simulink model "quadrotor_adaptive_control"  (R2025b)
settings: Solver=ode4  StartTime=0.0  StopTime=150  FixedStep=0.001  MaxStep=1e-3  RelTol=1e-6
values from neighbouring files (symbols this model uses):
  pi_hat0 = [0.899; 0.009; 0.009; 0.015]    [pi_hat_init.m]
undefined symbols (not defined in the file or in its folder): F, Light, MIL
libraries: simulink x5, aerolibwind2 x3
(part 1 of 2)
settings Model: Creator=Marcus  LastModifiedBy=Marcus
settings SolverCC: ZeroCrossAlgorithm=Adaptive
settings DataIOCC: Refine=5
settings DebuggingCC: MaskedZcDiagnostic=none  IgnoredZcDiagnostic=none

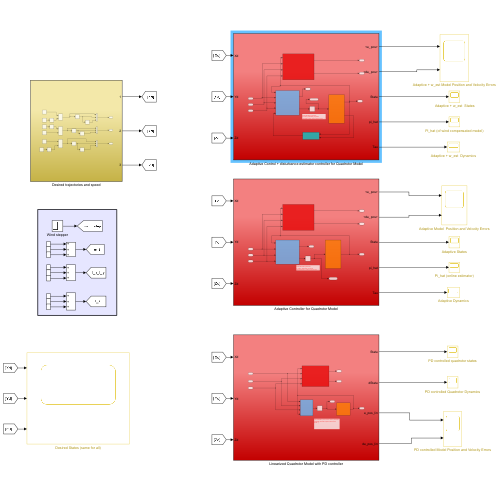
[thumbnail: Simulink's stored preview of the top-level diagram]
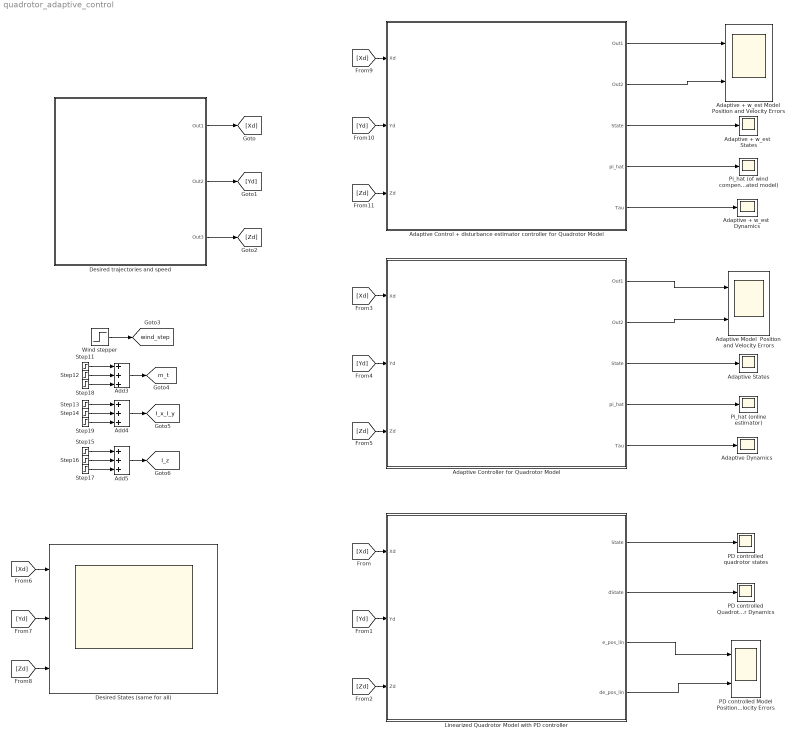
== system quadrotor_adaptive_control ==
  " Adaptive + w_est  States" : Scope
      settings: ActiveDisplayYMinimum=-16.300355765094039  ActiveDisplayYMaximum=35.268121644777928  DataLoggingVariableName=ScopeData9
  Adaptive + w_est  Dynamics : Scope
      settings: ActiveDisplayYMinimum=-3.5572864670508944  ActiveDisplayYMaximum=4.821971659312168  DataLoggingVariableName=ScopeData6
  Adaptive + w_est Model Position and Velocity Errors : Scope  NumInputPorts=2
      settings: ActiveDisplayYMinimum=-0.49516573839944322  ActiveDisplayYMaximum=0.3279252812181247  DataLoggingVariableName=ScopeData7
  Adaptive Control + disturbance estimator controller for Quadrotor Model : Subsystem
  Adaptive Controller for Quadrotor Model : Subsystem
  Adaptive Dynamics : Scope
      settings: ActiveDisplayYMinimum=-0.23880128032010212  ActiveDisplayYMaximum=0.18338732165681021  DataLoggingVariableName=ScopeData2
  Adaptive Model  Position and Velocity Errors : Scope  NumInputPorts=2
      settings: ActiveDisplayYMinimum=-0.24580483450326776  ActiveDisplayYMaximum=0.48785875848156551  DataLoggingVariableName=ScopeData3
  Adaptive States : Scope
      settings: ActiveDisplayYMinimum=-130.48583470390469  ActiveDisplayYMaximum=721.89809496547809
  Add3 : Sum  Inputs=+++
  Add4 : Sum  Inputs=+++
  Add5 : Sum  Inputs=+++
  Desired States (same for all) : Scope  NumInputPorts=3
      settings: ActiveDisplayYMinimum=-80.393154494146742  ActiveDisplayYMaximum=268.39207033687438
  Desired trajectories and speed : Subsystem
  Linearized Quadrotor Model with PD controller : Subsystem
  PD controlled Model Position and Velocity Errors : Scope  NumInputPorts=2
      settings: ActiveDisplayYMinimum=-1.1379166870147581  ActiveDisplayYMaximum=1.3439227788194077  DataLoggingVariableName=ScopeData8
  PD controlled Quadrotor Dynamics : Scope
      settings: ActiveDisplayYMinimum=-12.548402884641092  ActiveDisplayYMaximum=10.307273643056192  DataLoggingVariableName=ScopeData4
  PD controlled quadrotor states : Scope
      settings: ActiveDisplayYMinimum=-85.7969690316985  ActiveDisplayYMaximum=661.47891308235489  DataLoggingVariableName=ScopeData5
  Pi_hat (of wind compensated model) : Scope
      settings: ActiveDisplayYMinimum=1.5892477620700283  ActiveDisplayYMaximum=2.69868157713973  DataLoggingVariableName=pi_hat1  DataLoggingSaveFormat=Array
  Pi_hat (online estimator) : Scope
      settings: ActiveDisplayYMinimum=0.15390009207158523  ActiveDisplayYMaximum=0.19714737045984923  DataLoggingVariableName=pi_hat  DataLoggingSaveFormat=Array
  Step11 : Step  Time=50  Before=0.899  After=0.899+0.8  SampleTime=0
  Step12 : Step  Time=100  After=0.3  SampleTime=0
  Step13 : Step  Time=50  Before=0.009  After=0.009+0.002  SampleTime=0
  Step14 : Step  Time=100  After=0.28e-4  SampleTime=0
  Step15 : Step  Time=50  Before=0.015  After=0.015+0.15e-3*rand  SampleTime=0
  Step16 : Step  Time=100  After=0.2e-3  SampleTime=0
  Step17 : Step  Time=250  After=-0.12e-3  SampleTime=0
  Step18 : Step  Time=300  After=-0.2  SampleTime=0
  Step19 : Step  Time=240  After=-0.08e-4  SampleTime=0
  Wind stepper : Step  Time=85  SampleTime=0
  tag scope: I_x_I_y=global, I_z=global, m_t=global, wind_step=global
  wires:
  Linearized Quadrotor Model with PD controller/1(State) -> PD controlled quadrotor states/1
  Linearized Quadrotor Model with PD controller/2(dState) -> PD controlled Quadrotor Dynamics/1
  [Xd] -> Linearized Quadrotor Model with PD controller/1(Xd)
  [Yd] -> Linearized Quadrotor Model with PD controller/2(Yd)
  [Zd] -> Linearized Quadrotor Model with PD controller/3(Zd)
  [Xd] -> Adaptive Controller for Quadrotor Model/1(Xd)
  [Yd] -> Adaptive Controller for Quadrotor Model/2(Yd)
  [Zd] -> Adaptive Controller for Quadrotor Model/3(Zd)
  Adaptive Controller for Quadrotor Model/4(pi_hat) -> Pi_hat (online estimator)/1
  Adaptive Controller for Quadrotor Model/3(State) -> Adaptive States/1
  Adaptive Controller for Quadrotor Model/5(Tau) -> Adaptive Dynamics/1
  Adaptive Controller for Quadrotor Model/1(Out1) -> Adaptive Model  Position and Velocity Errors/1
  Adaptive Controller for Quadrotor Model/2(Out2) -> Adaptive Model  Position and Velocity Errors/2
  [Xd] -> Desired States (same for all)/1
  [Yd] -> Desired States (same for all)/2
  [Zd] -> Desired States (same for all)/3
  Linearized Quadrotor Model with PD controller/3(e_pos_lin) -> PD controlled Model Position and Velocity Errors/1
  Linearized Quadrotor Model with PD controller/4(de_pos_lin) -> PD controlled Model Position and Velocity Errors/2
  Adaptive Control + disturbance estimator controller for Quadrotor Model/5(Tau) -> Adaptive + w_est  Dynamics/1
  Adaptive Control + disturbance estimator controller for Quadrotor Model/4(pi_hat) -> Pi_hat (of wind compensated model)/1
  Adaptive Control + disturbance estimator controller for Quadrotor Model/2(Out2) -> Adaptive + w_est Model Position and Velocity Errors/2
  Adaptive Control + disturbance estimator controller for Quadrotor Model/1(Out1) -> Adaptive + w_est Model Position and Velocity Errors/1
  [Yd] -> Adaptive Control + disturbance estimator controller for Quadrotor Model/2(Yd)
  [Xd] -> Adaptive Control + disturbance estimator controller for Quadrotor Model/1(Xd)
  Adaptive Control + disturbance estimator controller for Quadrotor Model/3(State) -> " Adaptive + w_est  States"/1
  [Zd] -> Adaptive Control + disturbance estimator controller for Quadrotor Model/3(Zd)
  Wind stepper/1 -> [wind_step]
  Step16/1 -> Add5/2
  Step14/1 -> Add4/2
  Step11/1 -> Add3/1
  Step19/1 -> Add4/3
  Add4/1 -> [I_x_I_y]
  Step13/1 -> Add4/1
  Step18/1 -> Add3/3
  Add3/1 -> [m_t]
  Add5/1 -> [I_z]
  Step12/1 -> Add3/2
  Step15/1 -> Add5/1
  Step17/1 -> Add5/3
  Desired trajectories and speed/1(Out1) -> [Xd]
  Desired trajectories and speed/2(Out2) -> [Yd]
  Desired trajectories and speed/3(Out3) -> [Zd]

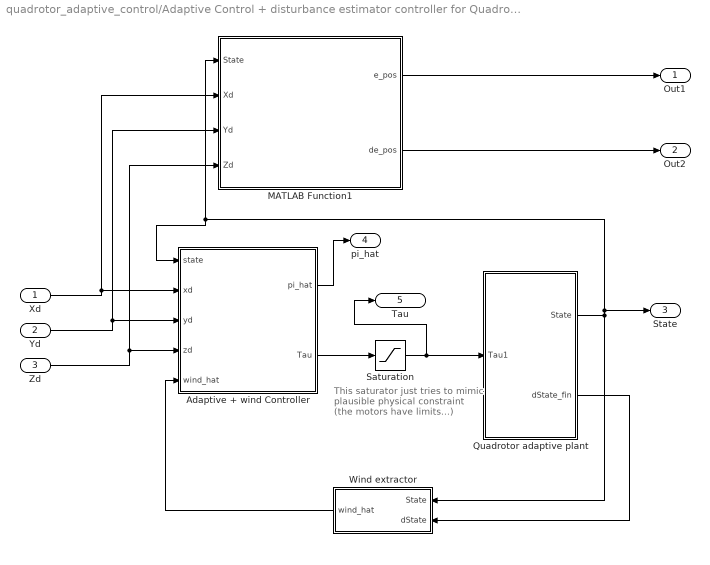
== system quadrotor_adaptive_control/Adaptive Control + disturbance estimator controller for Quadrotor Model ==
  note: This saturator just tries
      | to mimic plausible physical
      | constraint (the motors have limits...)
  Xd : Inport
  Yd : Inport  Port=2
  Zd : Inport  Port=3
  Adaptive + wind Controller : Subsystem
  MATLAB Function1 : MATLAB Function  TreatAsAtomicUnit=on
  Quadrotor adaptive plant : Subsystem
  Saturation : Saturate  UpperLimit=[25;0.8;0.8;0.10]  LowerLimit=[0;-0.8;-0.8;-0.10]
  Wind extractor : Subsystem
  Out1 : Outport
  Out2 : Outport  Port=2
  State : Outport  Port=3
  pi_hat : Outport  Port=4
  Tau : Outport  Port=5
  wires:
  Zd/1 -> MATLAB Function1/4(Zd), Adaptive + wind Controller/4(zd)
  Xd/1 -> MATLAB Function1/2(Xd), Adaptive + wind Controller/2(xd)
  Adaptive + wind Controller/1(pi_hat) -> pi_hat/1
  Yd/1 -> MATLAB Function1/3(Yd), Adaptive + wind Controller/3(yd)
  MATLAB Function1/2(de_pos) -> Out2/1
  MATLAB Function1/1(e_pos) -> Out1/1
  Quadrotor adaptive plant/1(State) -> State/1, MATLAB Function1/1(State), Adaptive + wind Controller/1(state), Wind extractor/1(State)
  Adaptive + wind Controller/2(Tau) -> Saturation/1
  Quadrotor adaptive plant/2(dState_fin) -> Wind extractor/2(dState)
  Wind extractor/1(wind_hat) -> Adaptive + wind Controller/5(wind_hat)
  Saturation/1 -> Tau/1, Quadrotor adaptive plant/1(Tau1)

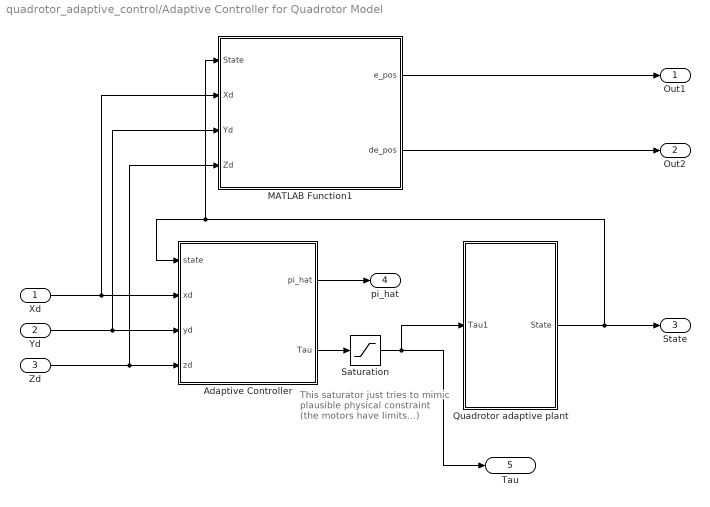
== system quadrotor_adaptive_control/Adaptive Controller for Quadrotor Model ==
  note: This saturator just tries
      | to mimic plausible physical
      | constraint (the motors have limits...)
  Xd : Inport
  Yd : Inport  Port=2
  Zd : Inport  Port=3
  Adaptive Controller : Subsystem
  MATLAB Function1 : MATLAB Function  TreatAsAtomicUnit=on
  Quadrotor adaptive plant : Subsystem
  Saturation : Saturate  UpperLimit=[25;0.8;0.8;0.10]  LowerLimit=[0;-0.8;-0.8;-0.10]
  Out1 : Outport
  Out2 : Outport  Port=2
  State : Outport  Port=3
  pi_hat : Outport  Port=4
  Tau : Outport  Port=5
  wires:
  Zd/1 -> MATLAB Function1/4(Zd), Adaptive Controller/4(zd)
  Adaptive Controller/2(Tau) -> Saturation/1
  Xd/1 -> MATLAB Function1/2(Xd), Adaptive Controller/2(xd)
  Adaptive Controller/1(pi_hat) -> pi_hat/1
  Yd/1 -> Adaptive Controller/3(yd), MATLAB Function1/3(Yd)
  MATLAB Function1/2(de_pos) -> Out2/1
  MATLAB Function1/1(e_pos) -> Out1/1
  Quadrotor adaptive plant/1(State) -> State/1, MATLAB Function1/1(State), Adaptive Controller/1(state)
  Saturation/1 -> Quadrotor adaptive plant/1(Tau1), Tau/1

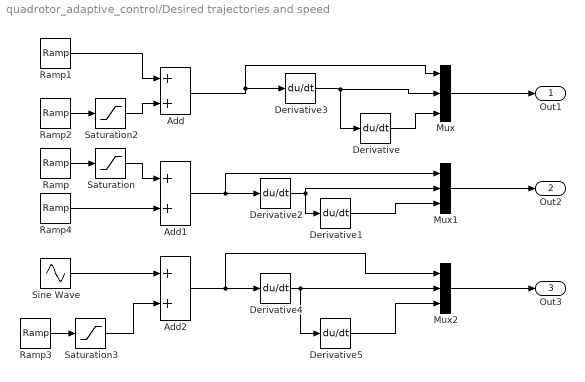
== system quadrotor_adaptive_control/Desired trajectories and speed ==
  Add : Sum
  Add1 : Sum
  Add2 : Sum
  Derivative{,1..5} (6 alike) : Derivative  CoefficientInTFapproximation=1e6
  Mux : Mux  Inputs=3
  Mux1 : Mux  Inputs=3
  Mux2 : Mux  Inputs=3
  Ramp : simulink/Sources/Ramp  slope=1.2  start=0  InitialOutput=0
  Ramp1 : simulink/Sources/Ramp  slope=0.3  start=0  InitialOutput=0
  Ramp2 : simulink/Sources/Ramp  slope=-1.2  start=65  InitialOutput=0
  Ramp3 : simulink/Sources/Ramp  slope=.4  start=70  InitialOutput=0
  Ramp4 : simulink/Sources/Ramp  slope=.2  start=20  InitialOutput=0
  Saturation : Saturate  UpperLimit=15  LowerLimit=0
  Saturation2 : Saturate  UpperLimit=0  LowerLimit=-5
  Saturation3 : Saturate  UpperLimit=3  LowerLimit=0
  Sine Wave : Sin  Bias=2  Frequency=0.5  SampleTime=0
  Out1 : Outport
  Out2 : Outport  Port=2
  Out3 : Outport  Port=3
  wires:
  Ramp/1 -> Saturation/1
  Add2/1 -> Derivative4/1, Mux2/1
  Saturation3/1 -> Add2/2
  Saturation/1 -> Add1/1
  Mux1/1 -> Out2/1
  Derivative4/1 -> Mux2/2, Derivative5/1
  Sine Wave/1 -> Add2/1
  Mux/1 -> Out1/1
  Mux2/1 -> Out3/1
  Ramp2/1 -> Saturation2/1
  Derivative5/1 -> Mux2/3
  Ramp1/1 -> Add/1
  Derivative/1 -> Mux/3
  Add/1 -> Mux/1, Derivative3/1
  Saturation2/1 -> Add/2
  Ramp3/1 -> Saturation3/1
  Derivative3/1 -> Mux/2, Derivative/1
  Ramp4/1 -> Add1/2
  Derivative1/1 -> Mux1/3
  Add1/1 -> Derivative2/1, Mux1/1
  Derivative2/1 -> Mux1/2, Derivative1/1

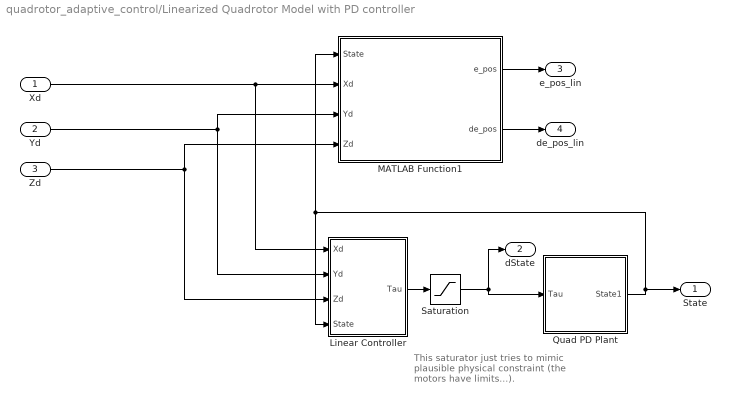
== system quadrotor_adaptive_control/Linearized Quadrotor Model with PD controller ==
  note: This saturator just tries to mimic plausible physical constraint (the motors have limits...).
  Xd : Inport
  Yd : Inport  Port=2
  Zd : Inport  Port=3
  Linear Controller : Subsystem
  MATLAB Function1 : MATLAB Function  TreatAsAtomicUnit=on
  Quad PD Plant : Subsystem
  Saturation : Saturate  UpperLimit=[25-8.82;0.8;0.8;0.10]  LowerLimit=[-8.82; -0.8;-0.8;-0.10]
  State : Outport
  dState : Outport  Port=2
  e_pos_lin : Outport  Port=3
  de_pos_lin : Outport  Port=4
  wires:
  Yd/1 -> Linear Controller/2(Yd), MATLAB Function1/3(Yd)
  Zd/1 -> Linear Controller/3(Zd), MATLAB Function1/4(Zd)
  Xd/1 -> Linear Controller/1(Xd), MATLAB Function1/2(Xd)
  MATLAB Function1/1(e_pos) -> e_pos_lin/1
  MATLAB Function1/2(de_pos) -> de_pos_lin/1
  Quad PD Plant/1(State1) -> Linear Controller/4(State), MATLAB Function1/1(State), State/1
  Linear Controller/1(Tau) -> Saturation/1
  Saturation/1 -> Quad PD Plant/1(Tau), dState/1

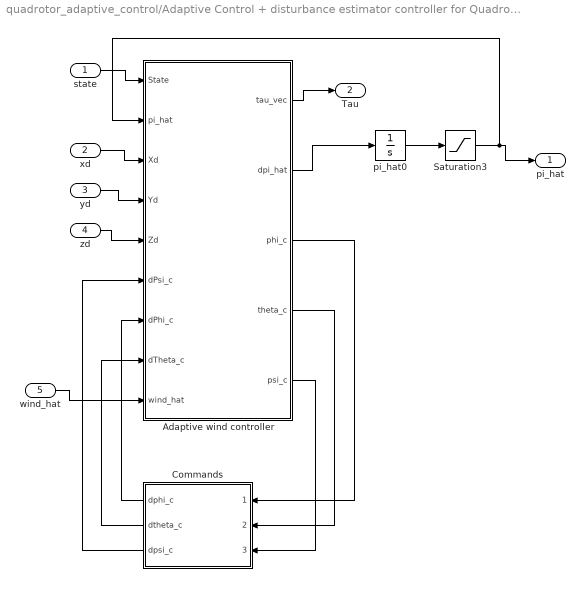
== system quadrotor_adaptive_control/Adaptive Control + disturbance estimator controller for Quadrotor Model/Adaptive + wind Controller ==
  state : Inport
  xd : Inport  Port=2
  yd : Inport  Port=3
  zd : Inport  Port=4
  wind_hat : Inport  Port=5
  Adaptive wind controller : MATLAB Function  TreatAsAtomicUnit=on
  "Commands " : Subsystem
  Saturation3 : Saturate  UpperLimit=[2.5;0.02; 0.02;0.02]  LowerLimit="[0.1; 0.001; 0.001;  0.002]"
  pi_hat0 : Integrator  InitialCondition=pi_hat0
  pi_hat : Outport
  Tau : Outport  Port=2
  wires:
  Adaptive wind controller/2(dpi_hat) -> pi_hat0/1
  Adaptive wind controller/1(tau_vec) -> Tau/1
  state/1 -> Adaptive wind controller/1(State)
  xd/1 -> Adaptive wind controller/3(Xd)
  yd/1 -> Adaptive wind controller/4(Yd)
  zd/1 -> Adaptive wind controller/5(Zd)
  "Commands "/3(dpsi_c) -> Adaptive wind controller/6(dPsi_c)
  "Commands "/1(dphi_c) -> Adaptive wind controller/7(dPhi_c)
  "Commands "/2(dtheta_c) -> Adaptive wind controller/8(dTheta_c)
  Adaptive wind controller/3(phi_c) -> "Commands "/1(1)
  Adaptive wind controller/4(theta_c) -> "Commands "/2(2)
  Adaptive wind controller/5(psi_c) -> "Commands "/3(3)
  pi_hat0/1 -> Saturation3/1
  Saturation3/1 -> pi_hat/1, Adaptive wind controller/2(pi_hat)
  wind_hat/1 -> Adaptive wind controller/9(wind_hat)

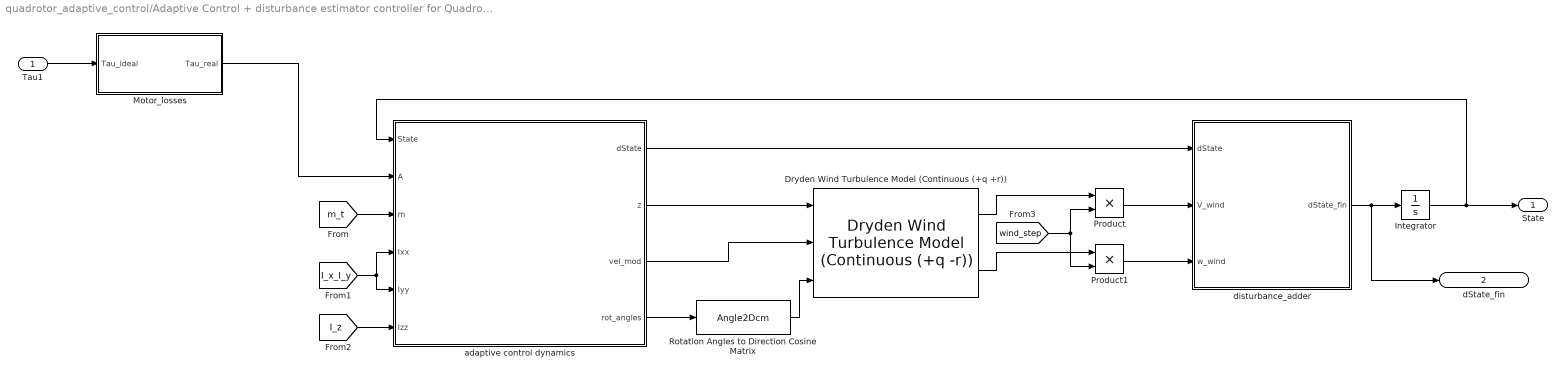
== system quadrotor_adaptive_control/Adaptive Control + disturbance estimator controller for Quadrotor Model/Quadrotor adaptive plant ==
  Tau1 : Inport
  Dryden Wind Turbulence Model (Continuous (+q +r)) : aerolibwind2/Dryden Wind Turbulence Model  (Continuous (+q -r))  units=Metric (MKS)  spec=MIL-F-8785C  model=Continuous Dryden (+q +r)  W20=10  Wdeg=0  TurbProb=10^-2 - Light  L_high=533.4  Wingspan=10  ts=0.1  Seed=[23341 23342 23343 23344]  T_on=on
      settings: LibrarySourceBlock=|
      | aerolibwind2/Dryden Wind Turbulence Model
      | (Continuous (+q +r))
  Integrator : Integrator  InitialCondition=zeros(12,1)
  Motor_losses : Subsystem
  Product : Product
  Product1 : Product
  Rotation Angles to Direction Cosine Matrix : Angle2Dcm  rotationOrder=ZXY
      settings: AttributesFormatString=Rotation Order: %<rotationOrder>
  adaptive control dynamics : MATLAB Function  TreatAsAtomicUnit=on
  disturbance_adder : MATLAB Function  TreatAsAtomicUnit=on
  State : Outport
  dState_fin : Outport  Port=2
  wires:
  Motor_losses/1(Tau_real) -> adaptive control dynamics/2(A)
  adaptive control dynamics/1(dState) -> disturbance_adder/1(dState)
  Rotation Angles to Direction Cosine Matrix/1 -> Dryden Wind Turbulence Model (Continuous (+q +r))/3
  adaptive control dynamics/2(z) -> Dryden Wind Turbulence Model (Continuous (+q +r))/1
  adaptive control dynamics/3(vel_mod) -> Dryden Wind Turbulence Model (Continuous (+q +r))/2
  adaptive control dynamics/4(rot_angles) -> Rotation Angles to Direction Cosine Matrix/1
  Integrator/1 -> State/1, adaptive control dynamics/1(State)
  disturbance_adder/1(dState_fin) -> dState_fin/1, Integrator/1
  Dryden Wind Turbulence Model (Continuous (+q +r))/1 -> Product/1
  Product/1 -> disturbance_adder/2(V_wind)
  Dryden Wind Turbulence Model (Continuous (+q +r))/2 -> Product1/1
  [wind_step] -> Product1/2, Product/2
  Product1/1 -> disturbance_adder/3(w_wind)
  Tau1/1 -> Motor_losses/1(Tau_ideal)
  [m_t] -> adaptive control dynamics/3(m)
  [I_x_I_y] -> adaptive control dynamics/5(Iyy), adaptive control dynamics/4(Ixx)
  [I_z] -> adaptive control dynamics/6(Izz)

== system quadrotor_adaptive_control/Adaptive Control + disturbance estimator controller for Quadrotor Model/Wind extractor ==
  State : Inport
  dState : Inport  Port=2
  MATLAB Function : MATLAB Function  TreatAsAtomicUnit=on
  Scope : Scope
      settings: ActiveDisplayYMinimum=-2.0656032479839856  ActiveDisplayYMaximum=0.38569203778728423  DataLoggingVariableName=ScopeData10
  wind extractor : Subsystem
  wind_hat : Outport
  wires:
  MATLAB Function/1(f_wnoise) -> wind extractor/1(fnoise)
  wind extractor/1(wind_hat) -> wind_hat/1, Scope/1
  dState/1 -> MATLAB Function/1(dState)
  State/1 -> MATLAB Function/2(State)

== system quadrotor_adaptive_control/Adaptive Controller for Quadrotor Model/Adaptive Controller ==
  state : Inport
  xd : Inport  Port=2
  yd : Inport  Port=3
  zd : Inport  Port=4
  Adaptive controller : MATLAB Function  TreatAsAtomicUnit=on
  "Commands " : Subsystem
  Saturation3 : Saturate  UpperLimit=[2.5;0.02; 0.02;0.02]  LowerLimit="[0.1; 0.001; 0.001;  0.002]"
  pi_hat0 : Integrator  InitialCondition=pi_hat0
  pi_hat : Outport
  Tau : Outport  Port=2
  wires:
  Adaptive controller/2(dpi_hat) -> pi_hat0/1
  Adaptive controller/1(tau_vec) -> Tau/1
  state/1 -> Adaptive controller/1(State)
  xd/1 -> Adaptive controller/3(Xd)
  yd/1 -> Adaptive controller/4(Yd)
  zd/1 -> Adaptive controller/5(Zd)
  "Commands "/3(dpsi_c) -> Adaptive controller/6(dPsi_c)
  "Commands "/1(dphi_c) -> Adaptive controller/7(dPhi_c)
  "Commands "/2(dtheta_c) -> Adaptive controller/8(dTheta_c)
  Adaptive controller/3(phi_c) -> "Commands "/1(1)
  Adaptive controller/4(theta_c) -> "Commands "/2(2)
  Adaptive controller/5(psi_c) -> "Commands "/3(3)
  pi_hat0/1 -> Saturation3/1
  Saturation3/1 -> Adaptive controller/2(pi_hat), pi_hat/1

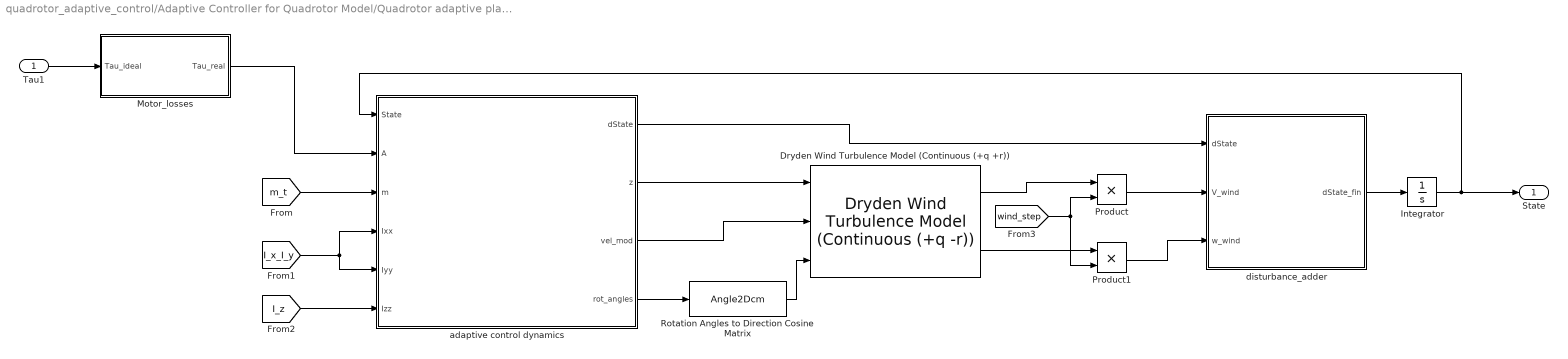
== system quadrotor_adaptive_control/Adaptive Controller for Quadrotor Model/Quadrotor adaptive plant ==
  Tau1 : Inport
  Dryden Wind Turbulence Model (Continuous (+q +r)) : aerolibwind2/Dryden Wind Turbulence Model  (Continuous (+q -r))  units=Metric (MKS)  spec=MIL-F-8785C  model=Continuous Dryden (+q +r)  W20=10  Wdeg=0  TurbProb=10^-2 - Light  L_high=533.4  Wingspan=10  ts=0.1  Seed=[23341 23342 23343 23344]  T_on=on
      settings: LibrarySourceBlock=|
      | aerolibwind2/Dryden Wind Turbulence Model
      | (Continuous (+q +r))
  Integrator : Integrator  InitialCondition=zeros(12,1)
  Motor_losses : Subsystem
  Product : Product
  Product1 : Product
  Rotation Angles to Direction Cosine Matrix : Angle2Dcm  rotationOrder=ZXY
      settings: AttributesFormatString=Rotation Order: %<rotationOrder>
  adaptive control dynamics : MATLAB Function  TreatAsAtomicUnit=on
  disturbance_adder : MATLAB Function  TreatAsAtomicUnit=on
  State : Outport
  wires:
  Motor_losses/1(Tau_real) -> adaptive control dynamics/2(A)
  adaptive control dynamics/1(dState) -> disturbance_adder/1(dState)
  Rotation Angles to Direction Cosine Matrix/1 -> Dryden Wind Turbulence Model (Continuous (+q +r))/3
  adaptive control dynamics/2(z) -> Dryden Wind Turbulence Model (Continuous (+q +r))/1
  adaptive control dynamics/3(vel_mod) -> Dryden Wind Turbulence Model (Continuous (+q +r))/2
  adaptive control dynamics/4(rot_angles) -> Rotation Angles to Direction Cosine Matrix/1
  Integrator/1 -> adaptive control dynamics/1(State), State/1
  disturbance_adder/1(dState_fin) -> Integrator/1
  Tau1/1 -> Motor_losses/1(Tau_ideal)
  [wind_step] -> Product1/2, Product/2
  Dryden Wind Turbulence Model (Continuous (+q +r))/1 -> Product/1
  Dryden Wind Turbulence Model (Continuous (+q +r))/2 -> Product1/1
  Product1/1 -> disturbance_adder/3(w_wind)
  Product/1 -> disturbance_adder/2(V_wind)
  [I_x_I_y] -> adaptive control dynamics/5(Iyy), adaptive control dynamics/4(Ixx)
  [I_z] -> adaptive control dynamics/6(Izz)
  [m_t] -> adaptive control dynamics/3(m)

== system quadrotor_adaptive_control/Linearized Quadrotor Model with PD controller/Linear Controller ==
  Xd : Inport
  Yd : Inport  Port=2
  Zd : Inport  Port=3
  State : Inport  Port=4
  "Commands " : Subsystem
  Linear Controller : MATLAB Function  TreatAsAtomicUnit=on
  Saturation1 : Saturate  UpperLimit=pi/9  LowerLimit=-pi/9
  Saturation2 : Saturate  UpperLimit=pi/9  LowerLimit=-pi/9
  Tau : Outport
  wires:
  Yd/1 -> Linear Controller/5(Yd)
  Zd/1 -> Linear Controller/6(Zd)
  Xd/1 -> Linear Controller/4(Xd)
  Linear Controller/1(Tau) -> Tau/1
  Linear Controller/2(phi_c) -> Saturation1/1
  "Commands "/2(dtheta_c) -> Linear Controller/3(dTheta_c)
  Linear Controller/3(theta_c) -> Saturation2/1
  State/1 -> Linear Controller/1(State)
  Saturation1/1 -> "Commands "/1(1)
  Saturation2/1 -> "Commands "/2(2)
  "Commands "/1(dphi_c) -> Linear Controller/2(dPhi_c)

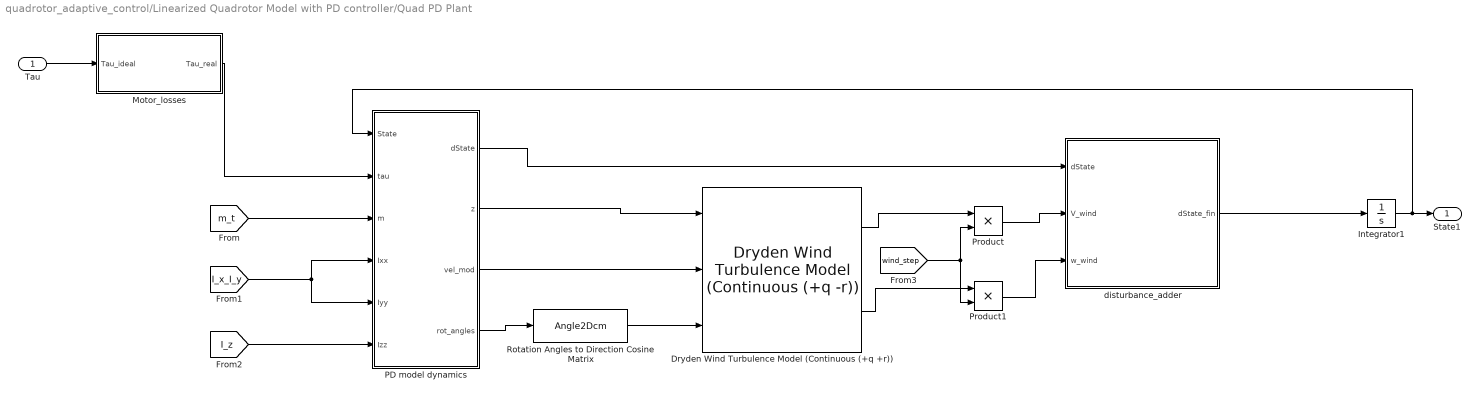
== system quadrotor_adaptive_control/Linearized Quadrotor Model with PD controller/Quad PD Plant ==
  Tau : Inport
  Dryden Wind Turbulence Model (Continuous (+q +r)) : aerolibwind2/Dryden Wind Turbulence Model  (Continuous (+q -r))  units=Metric (MKS)  spec=MIL-F-8785C  model=Continuous Dryden (+q +r)  W20=10  Wdeg=0  TurbProb=10^-2 - Light  L_high=533.4  Wingspan=10  ts=0.1  Seed=[23341 23342 23343 23344]  T_on=on
      settings: LibrarySourceBlock=|
      | aerolibwind2/Dryden Wind Turbulence Model
      | (Continuous (+q +r))
  Integrator1 : Integrator  InitialCondition=zeros(12,1)
  Motor_losses : Subsystem
  PD model dynamics : MATLAB Function  TreatAsAtomicUnit=on
  Product : Product
  Product1 : Product
  Rotation Angles to Direction Cosine Matrix : Angle2Dcm  rotationOrder=ZXY
      settings: AttributesFormatString=Rotation Order: %<rotationOrder>
  disturbance_adder : MATLAB Function  TreatAsAtomicUnit=on
  State1 : Outport
  wires:
  Motor_losses/1(Tau_real) -> PD model dynamics/2(tau)
  [m_t] -> PD model dynamics/3(m)
  [I_z] -> PD model dynamics/6(Izz)
  [I_x_I_y] -> PD model dynamics/5(Iyy), PD model dynamics/4(Ixx)
  PD model dynamics/3(vel_mod) -> Dryden Wind Turbulence Model (Continuous (+q +r))/2
  PD model dynamics/2(z) -> Dryden Wind Turbulence Model (Continuous (+q +r))/1
  Rotation Angles to Direction Cosine Matrix/1 -> Dryden Wind Turbulence Model (Continuous (+q +r))/3
  PD model dynamics/4(rot_angles) -> Rotation Angles to Direction Cosine Matrix/1
  disturbance_adder/1(dState_fin) -> Integrator1/1
  Integrator1/1 -> PD model dynamics/1(State), State1/1
  PD model dynamics/1(dState) -> disturbance_adder/1(dState)
  [wind_step] -> Product1/2, Product/2
  Product/1 -> disturbance_adder/2(V_wind)
  Dryden Wind Turbulence Model (Continuous (+q +r))/2 -> Product1/1
  Dryden Wind Turbulence Model (Continuous (+q +r))/1 -> Product/1
  Product1/1 -> disturbance_adder/3(w_wind)
  Tau/1 -> Motor_losses/1(Tau_ideal)

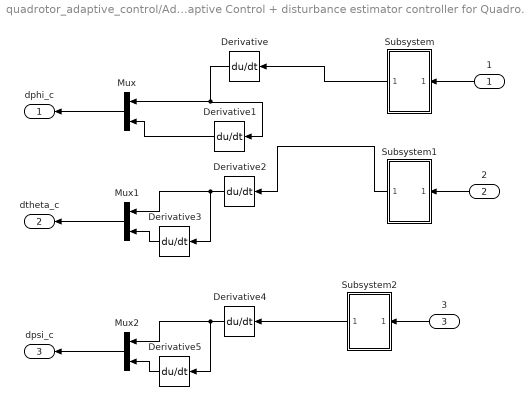
== system quadrotor_adaptive_control/Adaptive Control + disturbance estimator controller for Quadrotor Model/Adaptive + wind Controller/Commands  ==
  1 : Inport
  2 : Inport  Port=2
  3 : Inport  Port=3
  Derivative{,1..5} (6 alike) : Derivative  CoefficientInTFapproximation=1e6
  Mux : Mux  Inputs=2
  Mux1 : Mux  Inputs=2
  Mux2 : Mux  Inputs=2
  Subsystem : Subsystem
  Subsystem1 : Subsystem
  Subsystem2 : Subsystem
  dphi_c : Outport
  dtheta_c : Outport  Port=2
  dpsi_c : Outport  Port=3
  wires:
  Mux1/1 -> dtheta_c/1
  Mux/1 -> dphi_c/1
  Derivative2/1 -> Mux1/1, Derivative3/1
  Derivative3/1 -> Mux1/2
  Derivative/1 -> Derivative1/1, Mux/1
  1/1 -> Subsystem/1(In1)
  2/1 -> Subsystem1/1(In1)
  Derivative4/1 -> Mux2/1, Derivative5/1
  Mux2/1 -> dpsi_c/1
  Derivative5/1 -> Mux2/2
  3/1 -> Subsystem2/1(In1)
  Subsystem2/1(Out1) -> Derivative4/1
  Subsystem/1(Out1) -> Derivative/1
  Subsystem1/1(Out1) -> Derivative2/1
  Derivative1/1 -> Mux/2

== system quadrotor_adaptive_control/Adaptive Control + disturbance estimator controller for Quadrotor Model/Quadrotor adaptive plant/Motor_losses ==
  Tau_ideal : Inport
  20%_losses_for_motor1 : Subsystem
  20%_losses_for_motor2 : Subsystem
  20%_losses_for_motor3 : Subsystem
  20%_losses_for_motor4 : Subsystem
  Motor_loss : MATLAB Function  TreatAsAtomicUnit=on
  Tau_real : Outport
  wires:
  Motor_loss/1(Tau_real) -> Tau_real/1
  Tau_ideal/1 -> Motor_loss/1(Tau_ideal)
  20%_losses_for_motor1/1(f1_step) -> Motor_loss/2(f1_step)
  20%_losses_for_motor3/1(f3_step) -> Motor_loss/4(f3_step)
  20%_losses_for_motor2/1(f2_step) -> Motor_loss/3(f2_step)
  20%_losses_for_motor4/1(f4_step) -> Motor_loss/5(f4_step)

== system quadrotor_adaptive_control/Adaptive Control + disturbance estimator controller for Quadrotor Model/Wind extractor/wind extractor ==
  fnoise : Inport
  2 : TransferFcn  Numerator=1  Denominator=[0.1 1]
  Demux : Demux  Outputs=2
  Mux : Mux  Inputs=2
  Saturation : Saturate  UpperLimit=1.5  LowerLimit=-1.5
  Saturation1 : Saturate  UpperLimit=1.5  LowerLimit=-1.5
  wind acceleration extractor : TransferFcn  Numerator=1  Denominator=[0.1 1]
  wind_hat : Outport
  wires:
  Demux/1 -> wind acceleration extractor/1
  wind acceleration extractor/1 -> Saturation/1
  2/1 -> Saturation1/1
  Demux/2 -> 2/1
  Mux/1 -> wind_hat/1
  fnoise/1 -> Demux/1
  Saturation/1 -> Mux/1
  Saturation1/1 -> Mux/2

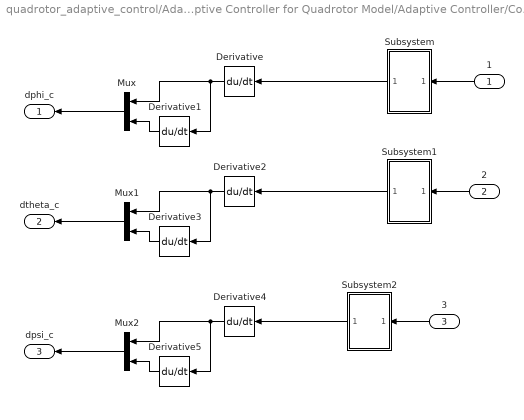
== system quadrotor_adaptive_control/Adaptive Controller for Quadrotor Model/Adaptive Controller/Commands  ==
  1 : Inport
  2 : Inport  Port=2
  3 : Inport  Port=3
  Derivative{,1..5} (6 alike) : Derivative  CoefficientInTFapproximation=1e6
  Mux : Mux  Inputs=2
  Mux1 : Mux  Inputs=2
  Mux2 : Mux  Inputs=2
  Subsystem : Subsystem
  Subsystem1 : Subsystem
  Subsystem2 : Subsystem
  dphi_c : Outport
  dtheta_c : Outport  Port=2
  dpsi_c : Outport  Port=3
  wires:
  Mux1/1 -> dtheta_c/1
  Mux/1 -> dphi_c/1
  Derivative1/1 -> Mux/2
  Derivative2/1 -> Mux1/1, Derivative3/1
  Derivative3/1 -> Mux1/2
  Derivative/1 -> Mux/1, Derivative1/1
  1/1 -> Subsystem/1(In1)
  2/1 -> Subsystem1/1(In1)
  Derivative4/1 -> Mux2/1, Derivative5/1
  Mux2/1 -> dpsi_c/1
  Derivative5/1 -> Mux2/2
  3/1 -> Subsystem2/1(In1)
  Subsystem/1(Out1) -> Derivative/1
  Subsystem1/1(Out1) -> Derivative2/1
  Subsystem2/1(Out1) -> Derivative4/1

== system quadrotor_adaptive_control/Adaptive Controller for Quadrotor Model/Quadrotor adaptive plant/Motor_losses ==
  Tau_ideal : Inport
  20%_losses_for_motor1 : Subsystem
  20%_losses_for_motor2 : Subsystem
  20%_losses_for_motor3 : Subsystem
  20%_losses_for_motor4 : Subsystem
  Motor_loss : MATLAB Function  TreatAsAtomicUnit=on
  Tau_real : Outport
  wires:
  Motor_loss/1(Tau_real) -> Tau_real/1
  Tau_ideal/1 -> Motor_loss/1(Tau_ideal)
  20%_losses_for_motor1/1(f1_step) -> Motor_loss/2(f1_step)
  20%_losses_for_motor3/1(f3_step) -> Motor_loss/4(f3_step)
  20%_losses_for_motor2/1(f2_step) -> Motor_loss/3(f2_step)
  20%_losses_for_motor4/1(f4_step) -> Motor_loss/5(f4_step)

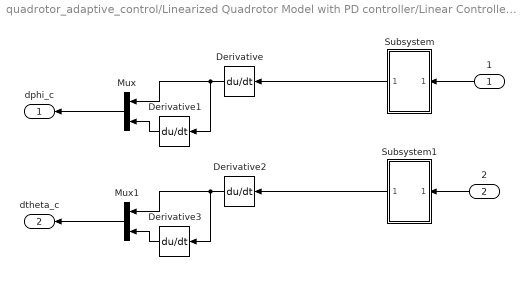
== system quadrotor_adaptive_control/Linearized Quadrotor Model with PD controller/Linear Controller/Commands  ==
  1 : Inport
  2 : Inport  Port=2
  Derivative{,1..3} (4 alike) : Derivative  CoefficientInTFapproximation=1e6
  Mux : Mux  Inputs=2
  Mux1 : Mux  Inputs=2
  Subsystem : Subsystem
  Subsystem1 : Subsystem
  dphi_c : Outport
  dtheta_c : Outport  Port=2
  wires:
  Subsystem1/1(Out1) -> Derivative2/1
  Subsystem/1(Out1) -> Derivative/1
  2/1 -> Subsystem1/1(In1)
  1/1 -> Subsystem/1(In1)
  Derivative/1 -> Derivative1/1, Mux/1
  Derivative3/1 -> Mux1/2
  Derivative2/1 -> Derivative3/1, Mux1/1
  Derivative1/1 -> Mux/2
  Mux/1 -> dphi_c/1
  Mux1/1 -> dtheta_c/1

== system quadrotor_adaptive_control/Linearized Quadrotor Model with PD controller/Quad PD Plant/Motor_losses ==
  Tau_ideal : Inport
  20%_losses_for_motor1 : Subsystem
  20%_losses_for_motor2 : Subsystem
  20%_losses_for_motor3 : Subsystem
  20%_losses_for_motor4 : Subsystem
  Motor_loss : MATLAB Function  TreatAsAtomicUnit=on
  Tau_real : Outport
  wires:
  Motor_loss/1(Tau_real) -> Tau_real/1
  Tau_ideal/1 -> Motor_loss/1(Tau_ideal)
  20%_losses_for_motor1/1(f1_step) -> Motor_loss/2(f1_step)
  20%_losses_for_motor3/1(f3_step) -> Motor_loss/4(f3_step)
  20%_losses_for_motor2/1(f2_step) -> Motor_loss/3(f2_step)
  20%_losses_for_motor4/1(f4_step) -> Motor_loss/5(f4_step)

== system quadrotor_adaptive_control/Adaptive Control + disturbance estimator controller for Quadrotor Model/Adaptive + wind Controller/Commands /Subsystem ==
  In1 : Inport
  Derivative4 : Derivative  CoefficientInTFapproximation=1e6
  Integrator1 : Integrator
  Out1 : Outport
  wires:
  Derivative4/1 -> Out1/1
  In1/1 -> Integrator1/1
  Integrator1/1 -> Derivative4/1

== system quadrotor_adaptive_control/Adaptive Control + disturbance estimator controller for Quadrotor Model/Adaptive + wind Controller/Commands /Subsystem1 ==
  In1 : Inport
  Derivative5 : Derivative  CoefficientInTFapproximation=1e6
  Integrator : Integrator
  Out1 : Outport
  wires:
  Derivative5/1 -> Out1/1
  In1/1 -> Integrator/1
  Integrator/1 -> Derivative5/1

== system quadrotor_adaptive_control/Adaptive Control + disturbance estimator controller for Quadrotor Model/Adaptive + wind Controller/Commands /Subsystem2 ==
  In1 : Inport
  Derivative5 : Derivative  CoefficientInTFapproximation=1e6
  Integrator : Integrator
  Out1 : Outport
  wires:
  Derivative5/1 -> Out1/1
  In1/1 -> Integrator/1
  Integrator/1 -> Derivative5/1

== system quadrotor_adaptive_control/Adaptive Control + disturbance estimator controller for Quadrotor Model/Quadrotor adaptive plant/Motor_losses/20%_losses_for_motor1 ==
  Add : Sum  Inputs=+++++
  Step : Step  Time=300  After=0.04  SampleTime=0
  Step1 : Step  Time=380  After=0.04  SampleTime=0
  Step2 : Step  Time=340  After=0.04  SampleTime=0
  Step3 : Step  Time=400  After=0.04  SampleTime=0
  Step4 : Step  Time=440  After=0.04  SampleTime=0
  f1_step : Outport
  wires:
  Step/1 -> Add/1
  Step3/1 -> Add/4
  Step1/1 -> Add/3
  Step2/1 -> Add/2
  Add/1 -> f1_step/1
  Step4/1 -> Add/5

== system quadrotor_adaptive_control/Adaptive Control + disturbance estimator controller for Quadrotor Model/Quadrotor adaptive plant/Motor_losses/20%_losses_for_motor2 ==
  Add : Sum  Inputs=+++++
  Step : Step  Time=300  After=0.04  SampleTime=0
  Step1 : Step  Time=380  After=0.04  SampleTime=0
  Step2 : Step  Time=340  After=0.04  SampleTime=0
  Step3 : Step  Time=400  After=0.04  SampleTime=0
  Step4 : Step  Time=440  After=0.04  SampleTime=0
  f2_step : Outport
  wires:
  Step/1 -> Add/1
  Step3/1 -> Add/4
  Step1/1 -> Add/3
  Step2/1 -> Add/2
  Add/1 -> f2_step/1
  Step4/1 -> Add/5

== system quadrotor_adaptive_control/Adaptive Control + disturbance estimator controller for Quadrotor Model/Quadrotor adaptive plant/Motor_losses/20%_losses_for_motor3 ==
  Add : Sum  Inputs=+++++
  Step : Step  Time=300  After=0.04  SampleTime=0
  Step1 : Step  Time=380  After=0.04  SampleTime=0
  Step2 : Step  Time=340  After=0.04  SampleTime=0
  Step3 : Step  Time=400  After=0.04  SampleTime=0
  Step4 : Step  Time=440  After=0.04  SampleTime=0
  f3_step : Outport
  wires:
  Step/1 -> Add/1
  Step3/1 -> Add/4
  Step1/1 -> Add/3
  Step2/1 -> Add/2
  Add/1 -> f3_step/1
  Step4/1 -> Add/5

== system quadrotor_adaptive_control/Adaptive Control + disturbance estimator controller for Quadrotor Model/Quadrotor adaptive plant/Motor_losses/20%_losses_for_motor4 ==
  Add : Sum  Inputs=+++++
  Step : Step  Time=300  After=0.04  SampleTime=0
  Step1 : Step  Time=380  After=0.04  SampleTime=0
  Step2 : Step  Time=340  After=0.04  SampleTime=0
  Step3 : Step  Time=400  After=0.04  SampleTime=0
  Step4 : Step  Time=440  After=0.04  SampleTime=0
  f4_step : Outport
  wires:
  Step/1 -> Add/1
  Step3/1 -> Add/4
  Step1/1 -> Add/3
  Step2/1 -> Add/2
  Add/1 -> f4_step/1
  Step4/1 -> Add/5

== system quadrotor_adaptive_control/Adaptive Controller for Quadrotor Model/Adaptive Controller/Commands /Subsystem ==
  In1 : Inport
  Derivative4 : Derivative  CoefficientInTFapproximation=1e6
  Integrator1 : Integrator
  Out1 : Outport
  wires:
  Derivative4/1 -> Out1/1
  In1/1 -> Integrator1/1
  Integrator1/1 -> Derivative4/1

== system quadrotor_adaptive_control/Adaptive Controller for Quadrotor Model/Adaptive Controller/Commands /Subsystem1 ==
  In1 : Inport
  Derivative5 : Derivative  CoefficientInTFapproximation=1e6
  Integrator : Integrator
  Out1 : Outport
  wires:
  Derivative5/1 -> Out1/1
  In1/1 -> Integrator/1
  Integrator/1 -> Derivative5/1

== system quadrotor_adaptive_control/Adaptive Controller for Quadrotor Model/Adaptive Controller/Commands /Subsystem2 ==
  In1 : Inport
  Derivative5 : Derivative  CoefficientInTFapproximation=1e6
  Integrator : Integrator
  Out1 : Outport
  wires:
  Derivative5/1 -> Out1/1
  In1/1 -> Integrator/1
  Integrator/1 -> Derivative5/1

== system quadrotor_adaptive_control/Adaptive Controller for Quadrotor Model/Quadrotor adaptive plant/Motor_losses/20%_losses_for_motor1 ==
  Add : Sum  Inputs=+++++
  Step : Step  Time=300  After=0.04  SampleTime=0
  Step1 : Step  Time=380  After=0.04  SampleTime=0
  Step2 : Step  Time=340  After=0.04  SampleTime=0
  Step3 : Step  Time=400  After=0.04  SampleTime=0
  Step4 : Step  Time=440  After=0.04  SampleTime=0
  f1_step : Outport
  wires:
  Step/1 -> Add/1
  Step3/1 -> Add/4
  Step1/1 -> Add/3
  Step2/1 -> Add/2
  Add/1 -> f1_step/1
  Step4/1 -> Add/5

== system quadrotor_adaptive_control/Adaptive Controller for Quadrotor Model/Quadrotor adaptive plant/Motor_losses/20%_losses_for_motor2 ==
  Add : Sum  Inputs=+++++
  Step : Step  Time=300  After=0.04  SampleTime=0
  Step1 : Step  Time=380  After=0.04  SampleTime=0
  Step2 : Step  Time=340  After=0.04  SampleTime=0
  Step3 : Step  Time=400  After=0.04  SampleTime=0
  Step4 : Step  Time=440  After=0.04  SampleTime=0
  f2_step : Outport
  wires:
  Step/1 -> Add/1
  Step3/1 -> Add/4
  Step1/1 -> Add/3
  Step2/1 -> Add/2
  Add/1 -> f2_step/1
  Step4/1 -> Add/5

== system quadrotor_adaptive_control/Adaptive Controller for Quadrotor Model/Quadrotor adaptive plant/Motor_losses/20%_losses_for_motor3 ==
  Add : Sum  Inputs=+++++
  Step : Step  Time=300  After=0.04  SampleTime=0
  Step1 : Step  Time=380  After=0.04  SampleTime=0
  Step2 : Step  Time=340  After=0.04  SampleTime=0
  Step3 : Step  Time=400  After=0.04  SampleTime=0
  Step4 : Step  Time=440  After=0.04  SampleTime=0
  f3_step : Outport
  wires:
  Step/1 -> Add/1
  Step3/1 -> Add/4
  Step1/1 -> Add/3
  Step2/1 -> Add/2
  Add/1 -> f3_step/1
  Step4/1 -> Add/5

== system quadrotor_adaptive_control/Adaptive Controller for Quadrotor Model/Quadrotor adaptive plant/Motor_losses/20%_losses_for_motor4 ==
  Add : Sum  Inputs=+++++
  Step : Step  Time=300  After=0.04  SampleTime=0
  Step1 : Step  Time=380  After=0.04  SampleTime=0
  Step2 : Step  Time=340  After=0.04  SampleTime=0
  Step3 : Step  Time=400  After=0.04  SampleTime=0
  Step4 : Step  Time=440  After=0.04  SampleTime=0
  f4_step : Outport
  wires:
  Step/1 -> Add/1
  Step3/1 -> Add/4
  Step1/1 -> Add/3
  Step2/1 -> Add/2
  Add/1 -> f4_step/1
  Step4/1 -> Add/5

== system quadrotor_adaptive_control/Linearized Quadrotor Model with PD controller/Linear Controller/Commands /Subsystem ==
  In1 : Inport
  Derivative4 : Derivative  CoefficientInTFapproximation=1e6
  Integrator1 : Integrator
  Out1 : Outport
  wires:
  Integrator1/1 -> Derivative4/1
  In1/1 -> Integrator1/1
  Derivative4/1 -> Out1/1

== system quadrotor_adaptive_control/Linearized Quadrotor Model with PD controller/Linear Controller/Commands /Subsystem1 ==
  In1 : Inport
  Derivative5 : Derivative  CoefficientInTFapproximation=1e6
  Integrator : Integrator
  Out1 : Outport
  wires:
  Integrator/1 -> Derivative5/1
  In1/1 -> Integrator/1
  Derivative5/1 -> Out1/1

== system quadrotor_adaptive_control/Linearized Quadrotor Model with PD controller/Quad PD Plant/Motor_losses/20%_losses_for_motor1 ==
  Add : Sum  Inputs=+++++
  Step : Step  Time=300  After=0.04  SampleTime=0
  Step1 : Step  Time=380  After=0.04  SampleTime=0
  Step2 : Step  Time=340  After=0.04  SampleTime=0
  Step3 : Step  Time=400  After=0.04  SampleTime=0
  Step4 : Step  Time=440  After=0.04  SampleTime=0
  f1_step : Outport
  wires:
  Step/1 -> Add/1
  Step3/1 -> Add/4
  Step1/1 -> Add/3
  Step2/1 -> Add/2
  Add/1 -> f1_step/1
  Step4/1 -> Add/5

== system quadrotor_adaptive_control/Linearized Quadrotor Model with PD controller/Quad PD Plant/Motor_losses/20%_losses_for_motor2 ==
  Add : Sum  Inputs=+++++
  Step : Step  Time=300  After=0.04  SampleTime=0
  Step1 : Step  Time=380  After=0.04  SampleTime=0
  Step2 : Step  Time=340  After=0.04  SampleTime=0
  Step3 : Step  Time=400  After=0.04  SampleTime=0
  Step4 : Step  Time=440  After=0.04  SampleTime=0
  f2_step : Outport
  wires:
  Step/1 -> Add/1
  Step3/1 -> Add/4
  Step1/1 -> Add/3
  Step2/1 -> Add/2
  Add/1 -> f2_step/1
  Step4/1 -> Add/5

== system quadrotor_adaptive_control/Linearized Quadrotor Model with PD controller/Quad PD Plant/Motor_losses/20%_losses_for_motor3 ==
  Add : Sum  Inputs=+++++
  Step : Step  Time=300  After=0.04  SampleTime=0
  Step1 : Step  Time=380  After=0.04  SampleTime=0
  Step2 : Step  Time=340  After=0.04  SampleTime=0
  Step3 : Step  Time=400  After=0.04  SampleTime=0
  Step4 : Step  Time=440  After=0.04  SampleTime=0
  f3_step : Outport
  wires:
  Step/1 -> Add/1
  Step3/1 -> Add/4
  Step1/1 -> Add/3
  Step2/1 -> Add/2
  Add/1 -> f3_step/1
  Step4/1 -> Add/5

== system quadrotor_adaptive_control/Linearized Quadrotor Model with PD controller/Quad PD Plant/Motor_losses/20%_losses_for_motor4 ==
  Add : Sum  Inputs=+++++
  Step : Step  Time=300  After=0.04  SampleTime=0
  Step1 : Step  Time=380  After=0.04  SampleTime=0
  Step2 : Step  Time=340  After=0.04  SampleTime=0
  Step3 : Step  Time=400  After=0.04  SampleTime=0
  Step4 : Step  Time=440  After=0.04  SampleTime=0
  f4_step : Outport
  wires:
  Step/1 -> Add/1
  Step3/1 -> Add/4
  Step1/1 -> Add/3
  Step2/1 -> Add/2
  Add/1 -> f4_step/1
  Step4/1 -> Add/5

== matlab function quadrotor_adaptive_control/Linearized Quadrotor Model with PD controller/MATLAB Function1 ==
  data: State input; e_pos output; Xd input; Yd input; Zd input; de_pos output
function [e_pos, de_pos] = error_calculator(State, Xd, Yd, Zd)
    
    % --- 1. STATE EXTRACTION ---
  
    x = State(1); y = State(2); z = State(3);
    u = State(4); v = State(5); w = State(6);
    
    phi = State(7); theta = State(8); psi = State(9);
    p = State(10); q = State(11); r = State(12);

    % --- 2. OUTER LOOP ERRORS
    % Standard convention: Error = Actual - Desired
    e_x = x - Xd(1); de_x = u - Xd(2);
    e_y = y - Yd(1); de_y = v - Yd(2);
    e_z = z - Zd(1); de_z = w - Zd(2);
    
    e_pos = [e_x; e_y; e_z];
    de_pos = [de_x; de_y; de_z];
end

== matlab function quadrotor_adaptive_control/Linearized Quadrotor Model with PD controller/Linear Controller/Linear Controller ==
  settings: updateMethod=DISCRETE
  data: State input; dPhi_c input; dTheta_c input; Tau output size=4; phi_c output size=1; theta_c output size=1; Xd input; Yd input; Zd input
function [Tau, phi_c, theta_c] = lin_controller(...
    State, ...
    dPhi_c, dTheta_c,...
    Xd, Yd, Zd)


    m     = 0.899;
    Ixx  = 0.009;
    Iyy   = 0.009;
    Izz   = 0.015; 

    %NOTE: IF WE UPDATED THE VALUES OF THE CONTROLLER WITH THE VALUES OF THE
    %      DYNAMIC MODEL (WHICH ARE CHANGING OVER TIME) THE LINEAR CONTROLLER
    %      WOULD BE UPDATED AS WELL AND WE WOULD NOT BE ABLE TO SEE THE
    %      POTENTIAL OF AN ADAPTIVE CONTROLLER!!!

    % --- CONSTANTS ---
    g = 9.81;
    psi_bar = 0; % Target yaw angle 

    % --- 1. STATE UNPACK ---
    x = State(1); y = State(2); z = State(3); 
    dx = State(4); dy = State(5); dz = State(6); 
    phi = State(7); theta = State(8); psi = State(9); 
    dphi = State(10); dtheta = State(11); dpsi = State(12);

    % --- 2. REFERENCE UNPACK ---
    x_d = Xd(1); dx_d = Xd(2); ddx_d = Xd(3);
    y_d = Yd(1); dy_d = Yd(2); ddy_d = Yd(3);
    z_d = Zd(1); dz_d = Zd(2); ddz_d = Zd(3);

    % Roll and Pitch feedforward from commands filter
    dphi_c = dPhi_c(1); ddphi_c = dPhi_c(2);
    dtheta_c = dTheta_c(1); ddtheta_c = dTheta_c(2);

    % --- 3. CONTROL GAINS ---
    lambda_pos = 3;
    kv_x = 2*lambda_pos; kp_x = lambda_pos^2;
    kv_y = 2*lambda_pos; kp_y = lambda_pos^2;
    kv_z = 2*lambda_pos; kp_z = lambda_pos^2;

    lambda_att = 6;
    kv_phi = 2*lambda_att; kp_phi = lambda_att^2;
    kv_theta = 2*lambda_att; kp_theta = lambda_att^2;
    kv_psi = 2*lambda_att; kp_psi = lambda_att^2;

    % --- 4. OUTER LOOP (Translational Control) ---
    C = 1/g * [sin(psi), -cos(psi); cos(psi), sin(psi) ] * ...
        [ ddx_d - kv_x * (dx - dx_d) - kp_x * (x - x_d); ...
          ddy_d - kv_y * (dy - dy_d) - kp_y * (y - y_d)];

    phi_c = C(1);
    theta_c = C(2);

    % --- 5. INNER LOOP (Attitude & Altitude Control) ---

    % Vertical thrust 
    deltaF = m * ( ddz_d - kv_z * (dz - dz_d) - kp_z * (z - z_d));
    

    % Torques
    tau_phi = Ixx * (ddphi_c - kv_phi * (dphi - dphi_c) - kp_phi * (phi - phi_c));
    tau_theta = Iyy * (ddtheta_c - kv_theta * (dtheta - dtheta_c) - kp_theta * (theta - theta_c));

    % Yaw control 
    tau_psi = Izz * (- kv_psi * dpsi - kp_psi * (psi - psi_bar));

    % --- 6. PACKED OUTPUT ---
    Tau = [deltaF; tau_phi; tau_theta; tau_psi];

end

== matlab function quadrotor_adaptive_control/Linearized Quadrotor Model with PD controller/Quad PD Plant/disturbance_adder ==
  data: dState input; V_wind input; w_wind input; dState_fin output size=12
function dState_fin = disturbance_adder(dState, V_wind, w_wind)
    % 1. NOMINAL dState UNPACKING
    dx0 = dState(1); dy0 = dState(2); dz0 = dState(3); % Velocità lineari
    du0 = dState(4); dv0 = dState(5); dw0 = dState(6); % Accelerazioni lineari
    dphi0 = dState(7); dtheta0 = dState(8); dpsi0 = dState(9); % Velocità angolari
    dp0 = dState(10); dq0 = dState(11); dr0 = dState(12); % Accelerazioni angolari
    
    % 2. V_wind and w_wind UNPACKING
    V_wind_x = V_wind(1); V_wind_y = V_wind(2); V_wind_z = V_wind(3);
    w_wind_phi = w_wind(1); w_wind_theta = w_wind(2); w_wind_psi = w_wind(3);
    
    % 3. Drag coefficients 
     Kd_lin = 0.6;  
     Kd_ang = 0.5;  
    
    % 4. Drag wind accelerations
    a_wind_x = Kd_lin * (V_wind_x - dx0);
    a_wind_y = Kd_lin * (V_wind_y - dy0);
    a_wind_z = Kd_lin * (V_wind_z - dz0);
    
    alpha_wind_phi = Kd_ang * (w_wind_phi - dphi0);
    alpha_wind_theta = Kd_ang * (w_wind_theta - dtheta0);
    alpha_wind_psi = Kd_ang * (w_wind_psi - dpsi0);
    
    % 5. Injenction of disturbance (on acceleration)
    du_fin = du0 + a_wind_x;
    dv_fin = dv0 + a_wind_y;
    dw_fin = dw0 + a_wind_z;
    
    dp_fin = dp0 + alpha_wind_phi;
    dq_fin = dq0 + alpha_wind_theta;
    dr_fin = dr0 + alpha_wind_psi;
    
    % 6. PACKING FINAL dState
    dState_fin = [dx0; dy0; dz0; du_fin; dv_fin; dw_fin; dphi0; dtheta0; dpsi0; dp_fin; dq_fin; dr_fin];
 
end

== matlab function quadrotor_adaptive_control/Adaptive Control + disturbance estimator controller for Quadrotor Model/Adaptive + wind Controller/Adaptive wind controller ==
  data: State input; tau_vec output size=[4 1]; pi_hat input; Xd input; Yd input; Zd input; dpi_hat output size=4; dPsi_c input; dPhi_c input; phi_c output size=1; theta_c output size=1; dTheta_c input; psi_c output; wind_hat input
function [tau_vec, dpi_hat, phi_c, theta_c, psi_c] = controller( ...
    State, pi_hat, Xd, Yd, Zd, dPsi_c, dPhi_c, dTheta_c, wind_hat)

    % ============================================================
    % ADAPTIVE + WIND-COMPENSATED CONTROLLER
    % wind compensation separated from parametric slotine-li adaptive control!!!
    % ============================================================

    % ---------- Tunable and adaptive control gains ----------
    Kd     = diag([2.0, 0.08, 0.08, 0.040]);
    Ks     = diag([5, 3.5, 3.5, 2]);
    Lambda = diag([5.0, 8.0, 8.0, 5.0]);
    Kpi    = diag([1.5, 0.003, 0.003, 0.008]);
    k_w = 1;

    % leakage 
    sigma_pi = diag([0.20, 0.002, 0.002, 0.004]);

    g  = 9.81;
    
    %nominal parameters 
    m0     = 0.899;
    Ixx0   = 0.009;
    Iyy0   = 0.009;
    Izz0   = 0.015;
    pi_nom = [m0; Ixx0; Iyy0; Izz0];
   
    % phi_max   = 0.35;  % [rad]    
    % theta_max = 0.35;    

    % ---------- 1) State extraction ----------
    x = State(1);   y = State(2);   z = State(3);
    u = State(4);   v = State(5);   w = State(6);
    phi = State(7); theta = State(8); psi = State(9);
    p = State(10);  q_rot = State(11); r = State(12);

    % ---------- 2) Desired references ----------
    x_d   = Xd(1);  dx_d   = Xd(2);  ddx_d   = Xd(3);
    y_d   = Yd(1);  dy_d   = Yd(2);  ddy_d   = Yd(3);
    z_d   = Zd(1);  dz_d   = Zd(2);  ddz_d   = Zd(3);

    % yaw fissato
    psi_d   = 0.0;
    dpsi_d  = 0.0;
    ddpsi_d = 0.0;

    % ---------- 3) Outer loop X-Y ----------
    e_x  = x - x_d;
    de_x = u - dx_d;

    e_y  = y - y_d;
    de_y = v - dy_d;

    % nominal controller acceleration with compensation of error
    a_x_nom = ddx_d - 8.0*de_x - 15.0*e_x;
    a_y_nom = ddy_d - 8.0*de_y - 15.0*e_y;

    %compensating wind with just nominal mass
    a_x = a_x_nom - k_w*wind_hat(1)/m0;
    a_y = a_y_nom - k_w*wind_hat(2)/m0;



    % ---------- 4) Kinematic inversion ----------

    phi_c   = (1/g) * (a_x * sin(psi_d) - a_y * cos(psi_d));
    theta_c = (1/g) * (a_x * cos(psi_d) + a_y * sin(psi_d));
    psi_c   = psi_d;

    %done externally
    % phi_c   = min(max(phi_c,   -phi_max),   phi_max);
    % theta_c = min(max(theta_c, -theta_max), theta_max);

    % ---------- 5) Reference derivatives ----------
    dphi_c   = dPhi_c(1);
    ddphi_c  = dPhi_c(2);

    dtheta_c  = dTheta_c(1);
    ddtheta_c = dTheta_c(2);

    % dPsi_c not used, yaw fixed
    

    % ---------- 6) Inner loop ----------
    e_z      = z - z_d;
    de_z     = w - dz_d;

    e_phi    = phi - phi_c;
    de_phi   = p - dphi_c;

    e_theta  = theta - theta_c;
    de_theta = q_rot - dtheta_c;

    e_psi    = psi - psi_d;
    de_psi   = r - dpsi_d;

    e_vec  = [e_z; e_phi; e_theta; e_psi];
    de_vec = [de_z; de_phi; de_theta; de_psi];
    ddq_d  = [ddz_d; ddphi_c; ddtheta_c; ddpsi_d];

    % sliding surface
    s = de_vec + Lambda * e_vec;

    % reference model
    dq_ref  = [dz_d; dphi_c; dtheta_c; dpsi_d] - Lambda * e_vec;
    ddq_ref = ddq_d - Lambda * de_vec;

    %not used, just to say it exists p_ref  = dq_ref(2);
    q_ref  = dq_ref(3);
    r_ref  = dq_ref(4);

    dp_ref = ddq_ref(2);
    dq_ref_att = ddq_ref(3);
    dr_ref = ddq_ref(4);

    ddz_ref = ddq_ref(1);

    % ---------- 7) Regressor ----------
    % pi_hat = [m; Ixx; Iyy; Izz]
    Y_z = ddz_ref + g;

    Y_att = [ dp_ref,      -q_rot*r_ref,   q_rot*r_ref;
              p*r_ref,      dq_ref_att,   -p*r_ref;
             -p*q_ref,      p*q_ref,       dr_ref ];

    Y = blkdiag(Y_z, Y_att);

    % ---------- 8) Control law ----------
    tau_vec = Y*pi_hat - Kd*e_vec - Ks*s;

    % ---------- 9) Adaptive law ----------
    s_norm = norm(s);

    if s_norm > 0.02
        dpi_hat = -Kpi * (Y.' * s) - sigma_pi * (pi_hat - pi_nom);
        % that sigma_pi term is just there to tell the system to stay at
        % to nominal values if variations are not too strong, just like an
        % " elastic spring" at fixed lenght...Really doesn't change much.
    else
        dpi_hat = -sigma_pi * (pi_hat - pi_nom);
        %pi_nom is pi_hat0, just a choice of a more explicit name that stands for nominal
    end
end

== matlab function quadrotor_adaptive_control/Adaptive Control + disturbance estimator controller for Quadrotor Model/MATLAB Function1 ==
  data: State input; e_pos output; Xd input; Yd input; Zd input; de_pos output
function [e_pos, de_pos] = error_calculator(State, Xd, Yd, Zd)
    
    % --- 1. STATE EXTRACTION ---
  
    x = State(1); y = State(2); z = State(3);
    u = State(4); v = State(5); w = State(6);
    
    phi = State(7); theta = State(8); psi = State(9);
    p = State(10); q = State(11); r = State(12);

    % --- 2. OUTER LOOP ERRORS
    % Standard convention: Error = Actual - Desired
    e_x = x - Xd(1); de_x = u - Xd(2);
    e_y = y - Yd(1); de_y = v - Yd(2);
    e_z = z - Zd(1); de_z = w - Zd(2);
    
    e_pos = [e_x; e_y; e_z];
    de_pos = [de_x; de_y; de_z];
end

== matlab function quadrotor_adaptive_control/Adaptive Control + disturbance estimator controller for Quadrotor Model/Quadrotor adaptive plant/adaptive control dynamics ==
  data: State input; dState output; A input; m input; Ixx input; Iyy input; Izz input; z output; vel_mod output; rot_angles output
function [dState, z, vel_mod, rot_angles] = adp_dynamics(State, A, m, Ixx, Iyy, Izz)
    % 1. STATE EXTRACTION
    x = State(1); y = State(2); z = State(3); 
    u = State(4); v = State(5); w = State(6); 
    phi = State(7); theta = State(8); psi = State(9); 
    p = State(10); q = State(11); r = State(12);
    
    % 2. CONTROL INPUT EXTRACTION (Total thrust and body torques)
    F = A(1); 
    tau_phi = A(2); tau_theta = A(3); tau_psi = A(4);
    
    g = 9.81;
    
    % Mass-normalized thrust (Specific force)
    f_norm = F / m; 
    
    % Definition of trigonometric functions for computational semplicity
    c_phi = cos(phi); s_phi = sin(phi); t_phi = tan(phi);
    c_theta = cos(theta); s_theta = sin(theta); 
    c_psi = cos(psi); s_psi = sin(psi);
    
    % Linear kinematics (Translational velocities)
    dx = u; dy = v; dz = w;
    
    % Translational dynamics (Linear accelerations using Z-X-Y convention)
    du = (s_theta * c_psi + s_phi * c_theta * s_psi) * f_norm;
    dv = (s_theta * s_psi - s_phi * c_theta * c_psi) * f_norm;
    dw = (c_phi * c_theta) * f_norm - g;
    
    % Angular kinematics 
    % Note: Derived for the Z-X-Y rotation sequence
    dphi = c_theta * p + s_theta * r;
    dtheta = t_phi * s_theta * p + q - t_phi * c_theta * r;
    dpsi = -(s_theta / c_phi) * p + (c_theta / c_phi) * r;
    
    % Angular dynamics (Euler's equations of motion for a rigid body)
    dp = (tau_phi - (Izz - Iyy) * q * r) / Ixx;
    dq = (tau_theta - (Ixx - Izz) * p * r) / Iyy;
    dr = (tau_psi - (Iyy - Ixx) * p * q) / Izz;
    
    % Vector assembly (State derivative packing)
    dState = [dx; dy; dz; du; dv; dw; dphi; dtheta; dpsi; dp; dq; dr];

    %modulus of speed
    vel_mod = sqrt(v^2+u^2+w^2)+ 0.01;

    %rotational angles packing
    rot_angles = [phi, theta, psi];

end
